simulink model "code_gen_HeadingHold"  (Simulink 7.5)
settings: Solver=FixedStepDiscrete  SolverMode=SingleTasking  StartTime=0.0  StopTime=10.0  FixedStep=0.01  RelTol=1e-3
InitFcn:
  | boat_constants
values from neighbouring files (symbols this model uses):
  figure8_waypoints = int32([ ... (first row only)    [boat_constants.m]
  OC2max = 49999    [boat_constants.m]    (also in simulation_constants.m)
  sampling_waypoints = int32([ ... (first row only)    [boat_constants.m]
  T_step = 0.01    [boat_constants.m]    (also in common.m)
  test_waypoints = int32([ ... (first row only)    [boat_constants.m]
undefined symbols (not defined in the file or in its folder): clearGpsData, clearSensorData, cpInitCommunications, DataEEInitAndClear, DataEEWrite, DiscIntNeverNeededParam, ecan1_buffered_transmit_matlab, ecan1_error_status_matlab, ecan1_init, ecan1_receive_matlab, getGpsData, getSensorData, Init_onlyOnce, Init_Reset, initCalibrationRange, initGps, processNewCommData, processNewGpsData, setHilMode, u1, u2, uart1EnqueueStateData, uart2EnqueueActuatorData, y1
libraries: simulink x85, dsPICdrivers x44, uSimLib x6, simulink_need_slupdate x4, aerolibconvert2 x2
(part 4 of 6)

== system code_gen_HeadingHold/Controller/Radio Control Inputs1/If Action Subsystem5 ==
  input : Inport  OutDataType=fixdt(1, 16)  OutScaling=2^0
  range : Inport  Port=2  OutDataType=fixdt(1, 16)  OutScaling=2^0
  Action Port : ActionPort  ActionType=else
  Add 8% center deadband : Subsystem
  Constant : Constant  Value=0  OutDataType=fixdt(1, 16)  OutScaling=2^0  OutDataTypeStr=Inherit: Inherit via back propagation
  Constant1 : Constant  Value=1000  OutDataType=fixdt(1, 16)  OutScaling=2^0  OutDataTypeStr=Inherit: Inherit via back propagation
  Data Type Conversion : DataTypeConversion  OutDataType=fixdt(1, 16)  OutScaling=2^0
  Data Type Conversion1 : DataTypeConversion  OutDataType=fixdt(1, 16)  OutScaling=2^0
  Demux : Demux  Outputs=2
  Map into range : Stateflow chart  TreatAsAtomicUnit=on
  Saturation : Saturate  UpperLimit=1000  LowerLimit=0  OutDataTypeMode=int16  OutDataType=fixdt(1, 16)  OutScaling=2^0  OutDataTypeStr=int16  RndMeth=Simplest
  Out1 : Outport  OutDataType=fixdt(1, 16)  OutScaling=2^0  InitialOutput=50
  wires:
  Constant1/1 -> Map into range/5(out_max)
  Constant/1 -> Map into range/4(out_min)
  Demux/1 -> Map into range/2(in_min)
  Demux/2 -> Map into range/3(in_max)
  range/1 -> Data Type Conversion1/1
  Map into range/1(mappedValue) -> Saturation/1
  Data Type Conversion/1 -> Map into range/1(val)
  Data Type Conversion1/1 -> Demux/1
  Saturation/1 -> Add 8% center deadband/1(In1)
  input/1 -> Data Type Conversion/1
  Add 8% center deadband/1(Out1) -> Out1/1

== system code_gen_HeadingHold/Controller/Radio Control Inputs1/Reset calibration range ==
  note: Reset the calibration range for each
      | channel before recalibration.
  Trigger : TriggerPort
  Constant1 : Constant  Value=[8000 8000]  OutDataType=fixdt(1, 16)  OutScaling=2^0  OutDataTypeStr=Inherit: Inherit via back propagation  SampleTime=Inf
  Data Store Write : DataStoreWrite  DataStoreName=throttleRange  SampleTime=-1
  Data Store Write1 : DataStoreWrite  DataStoreName=rudderRange  SampleTime=-1
  Data Store Write2 : DataStoreWrite  DataStoreName=trackRange  SampleTime=-1
  wires:
  Constant1/1 -> Data Store Write/1, Data Store Write1/1, Data Store Write2/1

== system code_gen_HeadingHold/Controller/Split trackCommand to singular commands/Countdown timer for trigger ==
  note: calibrationState is a uint8 with 3 states:
      | 0 is off,
      | 1 is timing down waiting to transition,
      | 2 is after a successful transition
  in : Inport
  Constant1 : Constant  OutDataTypeMode=uint8  OutDataType=fixdt(1, 16)  OutScaling=2^0  OutDataTypeStr=uint8  SampleTime=T_step
  Data Store Memory : DataStoreMemory  DataStoreName=timerState  ReadBeforeWriteMsg=warning  WriteAfterWriteMsg=warning  WriteAfterReadMsg=warning  DataType=uint8  OutDataType=fixdt(1, 16)  OutScaling=2^0  OutDataTypeStr=uint8
  Data Store Read : DataStoreRead  DataStoreName=timerState  SampleTime=T_step
  Data Type Conversion1 : DataTypeConversion  OutDataTypeMode=uint8  OutDataType=fixdt(1, 16)  OutScaling=2^0  OutDataTypeStr=uint8
  State transitions : Subsystem
  Timer : DiscreteIntegrator  gainval=100  ExternalReset=level  InitialConditionMode=State only (most efficient)  SampleTime=T_step  OutDataTypeMode=uint8  OutDataType=fixdt(1, 16)  OutScaling=2^0  OutDataTypeStr=uint8  RndMeth=Simplest  LimitOutput=on  UpperSaturationLimit=127  LowerSaturationLimit=0  ICPrevOutput=DiscIntNeverNeededParam  ICPrevScaledInput=DiscIntNeverNeededParam
  Unit Delay2 : UnitDelay  SampleTime=-1
  trigger : Outport  OutDataType=fixdt(1, 16)  OutScaling=2^0
  wires:
  Constant1/1 -> Timer/1
  Timer/1 -> State transitions/1(timer)
  Data Store Read/1 -> State transitions/3(timerState)
  Unit Delay2/1 -> Timer/2
  State transitions/1(startTimer) -> Unit Delay2/1
  in/1 -> Data Type Conversion1/1
  Data Type Conversion1/1 -> State transitions/2(level)
  State transitions/2(trigger) -> trigger/1

== system code_gen_HeadingHold/Controller/Split trackCommand to singular commands/Countdown timer for trigger1 ==
  note: calibrationState is a uint8 with 3 states:
      | 0 is off,
      | 1 is timing down waiting to transition,
      | 2 is after a successful transition
  in : Inport
  Constant1 : Constant  OutDataTypeMode=uint8  OutDataType=fixdt(1, 16)  OutScaling=2^0  OutDataTypeStr=uint8  SampleTime=T_step
  Data Store Memory : DataStoreMemory  DataStoreName=timerState2  ReadBeforeWriteMsg=warning  WriteAfterWriteMsg=warning  WriteAfterReadMsg=warning  DataType=uint8  OutDataType=fixdt(1, 16)  OutScaling=2^0  OutDataTypeStr=uint8
  Data Store Read : DataStoreRead  DataStoreName=timerState2  SampleTime=T_step
  Data Type Conversion1 : DataTypeConversion  OutDataTypeMode=uint8  OutDataType=fixdt(1, 16)  OutScaling=2^0  OutDataTypeStr=uint8
  State transitions : Subsystem
  Timer : DiscreteIntegrator  gainval=100  ExternalReset=level  InitialConditionMode=State only (most efficient)  SampleTime=T_step  OutDataTypeMode=uint8  OutDataType=fixdt(1, 16)  OutScaling=2^0  OutDataTypeStr=uint8  RndMeth=Simplest  LimitOutput=on  UpperSaturationLimit=127  LowerSaturationLimit=0  ICPrevOutput=DiscIntNeverNeededParam  ICPrevScaledInput=DiscIntNeverNeededParam
  Unit Delay2 : UnitDelay  SampleTime=-1
  trigger : Outport  OutDataType=fixdt(1, 16)  OutScaling=2^0
  wires:
  State transitions/2(trigger) -> trigger/1
  Data Type Conversion1/1 -> State transitions/2(level)
  in/1 -> Data Type Conversion1/1
  State transitions/1(startTimer) -> Unit Delay2/1
  Unit Delay2/1 -> Timer/2
  Data Store Read/1 -> State transitions/3(timerState)
  Timer/1 -> State transitions/1(timer)
  Constant1/1 -> Timer/1

== system code_gen_HeadingHold/Sensor Inputs/Estop detection/If Action Subsystem ==
  data : Inport  OutDataType=fixdt(1, 16)  OutScaling=2^0
  Action Port : ActionPort  ActionType=then
  Bitwise Operator : simulink/Logic and Bit Operations/Bitwise Operator  logicop=OR  UseBitMask=off  NumInputPorts=2  BitMask=bin2dec('11011001')  BitMaskRealWorld=Stored Integer
  Data Store Write : DataStoreWrite  DataStoreName=v_rpm  SampleTime=-1
  Data Type Conversion2 : DataTypeConversion  OutDataTypeMode=int16  OutDataType=fixdt(1, 16)  OutScaling=2^0  OutDataTypeStr=int16
  Data Type Conversion3 : DataTypeConversion  OutDataTypeMode=uint16  OutDataType=fixdt(1, 16)  OutScaling=2^0  OutDataTypeStr=uint16
  Demux : Demux  Outputs=2
  Selector : Selector  InputPortWidth=8  IndexOptions=Index vector (dialog)  Indices=[1 2]  OutputSizes=1
  Shift Arithmetic : simulink/Logic and Bit Operations/Shift Arithmetic  SystemSampleTime=-1  nBitShiftRight=-8  nBinPtShiftRight=0
  wires:
  Demux/1 -> Shift Arithmetic/1
  Shift Arithmetic/1 -> Bitwise Operator/1
  Demux/2 -> Bitwise Operator/2
  Selector/1 -> Data Type Conversion3/1
  Bitwise Operator/1 -> Data Type Conversion2/1
  data/1 -> Selector/1
  Data Type Conversion2/1 -> Data Store Write/1
  Data Type Conversion3/1 -> Demux/1

== system code_gen_HeadingHold/Sensor Inputs/Estop detection/Receive ECAN1 Message ==
  C Function Call [ecanFunctions.c] : dsPICdrivers/OTHERS/C Function Call  Tag=dsPIC_dsPIC_CFunctionCall  FctUpdate=Output Function  fctName='ecan1_receive_matlab'  INPUT_SIZE=1  INPUT1=--  INPUT2=--  INPUT3=--  OUTPUT_SIZE=4  OUTPUT1=uint32  SampleTime=ecan1_receive_sample_time  InputType=[ ]  OutputType=[ 6 ]  FctDeclaration=extern void ecan1_receive_matlab(uint32_T* y1);  FctCall=ecan1_receive_matlab(*%y1);  OrderingInOutPopup=None  FctStart=None  FctStart_Name=Init_onlyOnce  FctStart_Declaration=inline extern void Init_onlyOnce();  FctStart_Call=Init_onlyOnce();  FctInit=None  FctInit_Name=Init_Reset  FctInit_Declaration=inline extern void Init_Reset();  FctInit_Call=Init_Reset();  PinDigitalInput=[]  PinDigitalOutput=[]  AnalogueInput=[]
  Compare To Zero : simulink/Logic and Bit Operations/Compare To Zero  SystemSampleTime=-1  relop=~=  LogicOutDataTypeMode=uint8  ZeroCross=off
  Data Type Conversion : DataTypeConversion  OutDataTypeMode=boolean  OutDataType=sfix(16)  OutScaling=2^0  OutDataTypeStr=boolean
  Data Type Conversion1 : DataTypeConversion  OutDataTypeMode=uint32  OutDataType=fixdt(1, 16)  OutScaling=2^0  OutDataTypeStr=uint32
  Decompose uint64 : Subsystem
  Demux : Demux
  Extract Bits : simulink/Logic and Bit Operations/Extract Bits  SystemSampleTime=-1  bitsToExtract=Lower half  numBits=8  bitIdxRange=[0 7]  outScalingMode=Treat bit field as an integer
  Extract Bits1 : simulink/Logic and Bit Operations/Extract Bits  SystemSampleTime=-1  bitsToExtract=Range of bits  numBits=8  bitIdxRange=[16 23]  outScalingMode=Treat bit field as an integer
  Extract Bits2 : simulink/Logic and Bit Operations/Extract Bits  SystemSampleTime=-1  bitsToExtract=Range ending with least significant bit  numBits=29  bitIdxRange=[0 7]  outScalingMode=Treat bit field as an integer
  identifier : Outport  OutDataType=sfix(16)  OutScaling=2^0
  data : Outport  Port=2  OutDataType=sfix(16)  OutScaling=2^0
  remote : Outport  Port=3  OutDataType=sfix(16)  OutScaling=2^0
  new : Outport  Port=4  OutDataType=sfix(16)  OutScaling=2^0
  size : Outport  Port=5  OutDataType=sfix(16)  OutScaling=2^0
  wires:
  C Function Call [ecanFunctions.c]/1 -> Demux/1
  Demux/1 -> Extract Bits2/1, Compare To Zero/1
  Demux/3 -> Decompose uint64/2(high-order uint1)
  Demux/4 -> Extract Bits/1, Extract Bits1/1
  Data Type Conversion/1 -> remote/1
  Demux/2 -> Decompose uint64/1(low-order uint32)
  Extract Bits/1 -> Data Type Conversion/1
  Decompose uint64/1(uint8 array) -> data/1
  Extract Bits2/1 -> Data Type Conversion1/1
  Compare To Zero/1 -> new/1
  Extract Bits1/1 -> size/1
  Data Type Conversion1/1 -> identifier/1

== system code_gen_HeadingHold/Transmit actuator data/Package and Transmit Sensor Struct/Build HIL sentence ==
  data : Inport
  Bitwise Operator : simulink/Logic and Bit Operations/Bitwise Operator  logicop=XOR  UseBitMask=off  BitMask=bin2dec('11011001')  BitMaskRealWorld=Stored Integer
  Constant : Constant  Value=37  OutDataTypeMode=uint8  OutDataType=fixdt(1, 16)  OutScaling=2^0  OutDataTypeStr=uint8
  Constant1 : Constant  Value=38  OutDataTypeMode=uint8  OutDataType=fixdt(1, 16)  OutScaling=2^0  OutDataTypeStr=uint8
  Constant2 : Constant  Value=94  OutDataTypeMode=uint8  OutDataType=fixdt(1, 16)  OutScaling=2^0  OutDataTypeStr=uint8
  Constant3 : Constant  Value=38  OutDataTypeMode=uint8  OutDataType=fixdt(1, 16)  OutScaling=2^0  OutDataTypeStr=uint8
  Constant4 : Constant  Value=2  OutDataTypeMode=uint8  OutDataType=fixdt(1, 16)  OutScaling=2^0  OutDataTypeStr=uint8
  Mux2 : Mux  Inputs=3
  Pack : Stateflow chart  TreatAsAtomicUnit=on
  Probe : Probe  ProbeSampleTime=off  ProbeComplexSignal=off  ProbeWidthDataType=uint8
  sent : Outport
  wires:
  data/1 -> Probe/1, Mux2/3
  Constant/1 -> Pack/1(a)
  Constant1/1 -> Pack/2(b)
  Pack/1(y) -> sent/1
  Mux2/1 -> Bitwise Operator/1, Pack/3(c)
  Probe/1 -> Mux2/2
  Constant2/1 -> Pack/4(d)
  Constant3/1 -> Pack/5(e)
  Bitwise Operator/1 -> Pack/6(f)
  Constant4/1 -> Mux2/1

== system code_gen_HeadingHold/Controller/Auto/Manual Switch/Rudder calibration controller/Rudder Command ==
  note: Up and period are both defined to generate a 50% duty cycle PWM with
      | a period of 3ms.
  step : Inport
  dir : Inport  Port=2
  Bus Creator : BusCreator
  Constant1 : Constant  Value=.003*OC2max/.01  OutDataTypeMode=uint16  OutDataType=sfix(16)  OutScaling=2^0  OutDataTypeStr=uint16
  Constant3 : Constant  Value=0  OutDataTypeMode=boolean  OutDataType=sfix(16)  OutScaling=2^0  OutDataTypeStr=boolean
  Constant4 : Constant  Value=0  OutDataTypeMode=uint16  OutDataType=sfix(16)  OutScaling=2^0  OutDataTypeStr=uint16
  Shift Arithmetic : simulink/Logic and Bit Operations/Shift Arithmetic  SystemSampleTime=-1  nBitShiftRight=1  nBinPtShiftRight=0
  Switch : Switch  Criteria=u2 ~= 0  OutDataType=fixdt(1, 16)  OutScaling=2^0
  Switch1 : Switch  Criteria=u2 ~= 0  OutDataType=fixdt(1, 16)  OutScaling=2^0
  Command : Outport
  wires:
  step/1 -> Switch1/2, Switch/2
  Constant4/1 -> Switch1/3, Switch/3
  Switch1/1 -> Bus Creator/3  "up"
  Switch/1 -> Bus Creator/4  "period"
  Shift Arithmetic/1 -> Switch1/1
  Constant1/1 -> Switch/1, Shift Arithmetic/1
  Constant3/1 -> Bus Creator/1  "enable"
  Bus Creator/1 -> Command/1
  dir/1 -> Bus Creator/2  "direction"

== system code_gen_HeadingHold/Controller/Auto/Manual Switch/Rudder calibration controller/Throttle Command ==
  en : Inport
  Bus Creator : BusCreator
  Logical Operator : Logic  Operator=NOT  AllPortsSameDT=off  OutDataTypeMode=boolean  LogicDataType=fixdt(0, 8)  OutDataTypeStr=boolean
  Mux Everything : Subsystem
  command : Outport  OutDataType=sfix(16)  OutScaling=2^0
  wires:
  Mux Everything/3(size) -> Bus Creator/3  "size"
  Mux Everything/2(data) -> Bus Creator/2  "data"
  Mux Everything/1(iden) -> Bus Creator/1  "identifier"
  en/1 -> Logical Operator/1
  Bus Creator/1 -> command/1
  Logical Operator/1 -> Mux Everything/1(reset)
  Mux Everything/4(trig) -> Bus Creator/4  "trigger"

== system code_gen_HeadingHold/Controller/Autonomous Controller/Rudder Command/Heading Control ==
  note: Heading Error
  V_boat [m/s] : Inport  OutDataType=sfix(16)  OutScaling=2^0
  Psi desired [deg] : Inport  Port=2  OutDataType=sfix(16)  OutScaling=2^0
  Heading [deg] : Inport  Port=3  OutDataType=sfix(16)  OutScaling=2^0
  CrossTrack Error [m] : Inport  Port=4  OutDataType=sfix(16)  OutScaling=2^0
  Abs : Abs
  Angle Conversion : aerolibconvert2/Angle Conversion  SystemSampleTime=-1  IU=deg  OU=rad
  Angle Conversion1 : aerolibconvert2/Angle Conversion  SystemSampleTime=-1  IU=rad  OU=deg
  Constant : Constant  OutDataType=sfix(16)  OutScaling=2^0
  Divide : Product  Inputs=*/  OutDataType=sfix(16)  OutScaling=2^-10
  Fcn2 : Fcn  Expr=(u<-180)*360 + u + (u>180)*(-360)
  Kpsi : Gain  ParameterDataType=sfix(16)  ParameterScaling=2^0  OutDataType=sfix(16)  OutScaling=2^0
  MinMax : MinMax  Function=max  Inputs=2  OutDataType=sfix(16)  OutScaling=2^0
  Product : Product  OutDataType=sfix(16)  OutScaling=2^0  RndMeth=Zero
  Saturation : Saturate  UpperLimit=45  LowerLimit=-45
  Scope : Scope
      settings: SaveName=ScopeData4
  Sign : Signum
  Sum : Sum  Inputs=-+|  OutDataType=sfix(16)  OutScaling=2^0
  Terminator : Terminator
  delta_R [deg] : Outport  OutDataType=sfix(16)  OutScaling=2^0
  wires:
  Fcn2/1 -> Angle Conversion/1, Scope/1
  Angle Conversion/1 -> Kpsi/1
  V_boat [m/s]/1 -> Abs/1, Sign/1
  Product/1 -> Angle Conversion1/1
  Kpsi/1 -> Product/2
  Sign/1 -> Product/1
  Angle Conversion1/1 -> Divide/1
  Divide/1 -> Saturation/1
  Abs/1 -> MinMax/1
  Constant/1 -> MinMax/2
  Saturation/1 -> delta_R [deg]/1
  MinMax/1 -> Divide/2
  CrossTrack Error [m]/1 -> Terminator/1
  Psi desired [deg]/1 -> Sum/1
  Heading [deg]/1 -> Sum/2
  Sum/1 -> Fcn2/1

== system code_gen_HeadingHold/Controller/Autonomous Controller/State Keeper & Estimator/Ballast Estimator ==
  b : Inport
  Bus Selector1 : BusSelector  OutputSignals=position
  sensors_b : Outport
  wires:
  Bus Selector1/1 -> sensors_b/1  "<position>"
  b/1 -> Bus Selector1/1

== system code_gen_HeadingHold/Controller/Autonomous Controller/State Keeper & Estimator/GPS Estimator ==
  gps : Inport
  reset : Inport  Port=2  OutDataType=fixdt(1, 16)  OutScaling=2^0
  Add : Sum  OutDataType=fixdt(1, 16)  OutScaling=2^-10
  Bus Selector1 : BusSelector  OutputSignals=latitude,longitude,altitude,newData
  Calculate local position via velocity integral between true GPS updates : Stateflow chart  TreatAsAtomicUnit=on
  Discrete-Time Integrator4 : DiscreteIntegrator  ExternalReset=level  SampleTime=-1  OutDataType=fixdt(1, 16)  OutScaling=2^0  ICPrevOutput=DiscIntNeverNeededParam  ICPrevScaledInput=DiscIntNeverNeededParam
  Mux1 : Mux  Inputs=3
  Subsystem : Subsystem
  velocity : Outport
  pos : Outport  Port=2
  heading : Outport  Port=3
  lla : Outport  Port=4
  datetime : Outport  Port=5
  wires:
  Subsystem/1(velocity) -> velocity/1, Discrete-Time Integrator4/1
  Calculate local position via velocity integral between true GPS updates/1(localPosition) -> Add/1
  Calculate local position via velocity integral between true GPS updates/2(resetIntegrator) -> Discrete-Time Integrator4/2
  Mux1/1 -> Calculate local position via velocity integral between true GPS updates/1(latLonAlt)
  Bus Selector1/4 -> Calculate local position via velocity integral between true GPS updates/2(newData)  "<newData>"
  Bus Selector1/3 -> Mux1/3  "<altitude>"
  Bus Selector1/2 -> Mux1/2  "<longitude>"
  Bus Selector1/1 -> Mux1/1  "<latitude>"
  Add/1 -> pos/1
  Discrete-Time Integrator4/1 -> Add/2
  reset/1 -> Calculate local position via velocity integral between true GPS updates/3(reset)
  Subsystem/4(time) -> datetime/1
  Subsystem/3(pos) -> lla/1
  gps/1 -> Bus Selector1/1, Subsystem/1(gps)
  Subsystem/2(heading) -> heading/1

== system code_gen_HeadingHold/Controller/Autonomous Controller/State Keeper & Estimator/Rudder Estimator ==
  r : Inport
  sensors_r : Outport
  wires:
  r/1 -> sensors_r/1

== system code_gen_HeadingHold/Controller/Autonomous Controller/State Keeper & Estimator/Throttle Estimator ==
  t : Inport
  sensors_t : Outport
  wires:
  t/1 -> sensors_t/1

== system code_gen_HeadingHold/Controller/Autonomous Controller/Throttle Command/Mux Everything ==
  speed : Inport  OutDataType=sfix(16)  OutScaling=2^0
  disable : Inport  Port=2  OutDataType=sfix(16)  OutScaling=2^0
  enable : Inport  Port=3  OutDataType=sfix(16)  OutScaling=2^0
  Throttle : Inport  Port=4  OutDataType=sfix(16)  OutScaling=2^0
  0x300 : Constant  Value=768  OutDataTypeMode=uint32  OutDataType=sfix(16)  OutScaling=2^0  OutDataTypeStr=uint32
  0x301 : Constant  Value=769  OutDataTypeMode=uint32  OutDataType=sfix(16)  OutScaling=2^0  OutDataTypeStr=uint32
  Build speed command : Subsystem
  Disable motor : Constant  Value=[0 0 0 0 64 0]  OutDataTypeMode=uint8  OutDataType=sfix(16)  OutScaling=2^0  OutDataTypeStr=uint8
  Enable motor : Constant  Value=[0 0 0 0 32 0]  OutDataTypeMode=uint8  OutDataType=sfix(16)  OutScaling=2^0  OutDataTypeStr=uint8
  Logical Operator1 : Logic  Operator=OR  AllPortsSameDT=off  OutDataTypeMode=boolean  OutDataTypeStr=boolean
  Message Length1 : Probe  ProbeSampleTime=off  ProbeComplexSignal=off  ProbeWidthDataType=uint8
  Multiport Switch : MultiPortSwitch  zeroidx=off
  Multiport Switch1 : MultiPortSwitch  zeroidx=off
  Select data packet : Stateflow chart  TreatAsAtomicUnit=on
  Switch : Switch  Criteria=u2 ~= 0
  iden : Outport  OutDataType=sfix(16)  OutScaling=2^0
  data : Outport  Port=2  OutDataType=sfix(16)  OutScaling=2^0
  size : Outport  Port=3  OutDataType=sfix(16)  OutScaling=2^0
  trig : Outport  Port=4  OutDataType=sfix(16)  OutScaling=2^0
  wires:
  Build speed command/1(msg) -> Multiport Switch/4
  speed/1 -> Multiport Switch1/4
  Multiport Switch1/1 -> trig/1
  Select data packet/1(y) -> Multiport Switch1/1, Multiport Switch/1
  Logical Operator1/1 -> Switch/2
  enable/1 -> Multiport Switch1/3, Select data packet/2(en), Logical Operator1/2
  disable/1 -> Multiport Switch1/2, Select data packet/1(dis), Logical Operator1/1
  Switch/1 -> iden/1
  0x301/1 -> Switch/3
  0x300/1 -> Switch/1
  Message Length1/1 -> size/1
  Multiport Switch/1 -> data/1, Message Length1/1
  Throttle/1 -> Build speed command/1(CC)
  Disable motor/1 -> Multiport Switch/2
  Enable motor/1 -> Multiport Switch/3

== system code_gen_HeadingHold/Controller/Autonomous Controller/Throttle Command/Trigger Events ==
  RC Throttle : Inport  OutDataType=sfix(16)  OutScaling=2^0
  Reset : Inport  Port=2  OutDataType=sfix(16)  OutScaling=2^0
  Data Type Conversion1 : DataTypeConversion  OutDataTypeMode=boolean  OutDataType=sfix(16)  OutScaling=2^0  OutDataTypeStr=boolean
  Data Type Conversion2 : DataTypeConversion  OutDataTypeMode=boolean  OutDataType=sfix(16)  OutScaling=2^0  OutDataTypeStr=boolean
  Data Type Conversion3 : DataTypeConversion  OutDataTypeMode=boolean  OutDataType=sfix(16)  OutScaling=2^0  OutDataTypeStr=boolean
  Detect Change : simulink/Logic and Bit Operations/Detect Change  SystemSampleTime=-1  vinit=0
  Detect Fall Nonpositive : simulink/Logic and Bit Operations/Detect Fall Nonpositive  SystemSampleTime=-1  vinit=0
  Detect Rise Positive : simulink/Logic and Bit Operations/Detect Rise Positive  SystemSampleTime=-1  vinit=0
  Shift Arithmetic : simulink/Logic and Bit Operations/Shift Arithmetic  SystemSampleTime=-1  nBitShiftRight=2  nBinPtShiftRight=0
  Weighted Moving Average : simulink_need_slupdate/Weighted Moving Average  mgainval=[.5 .5]  vinit=0.0  samptime=-1  OutDataTypeStr=Inherit: Inherit via back propagation  OutDataType=sfix(16)  OutScaling=2^-10  DoSatur=off  GainDataType=uint(16)  MatRadixGroup=Best Precision: Matrix-wise  GainScaling=2^-10
  Change Speed : Outport  OutDataType=sfix(16)  OutScaling=2^0
  Disable : Outport  Port=2  OutDataType=sfix(16)  OutScaling=2^0
  Enable : Outport  Port=3  OutDataType=sfix(16)  OutScaling=2^0
  wires:
  Data Type Conversion1/1 -> Disable/1
  Data Type Conversion2/1 -> Enable/1
  Data Type Conversion3/1 -> Change Speed/1
  Detect Rise Positive/1 -> Data Type Conversion1/1
  Detect Fall Nonpositive/1 -> Data Type Conversion2/1
  Reset/1 -> Detect Rise Positive/1, Detect Fall Nonpositive/1
  Shift Arithmetic/1 -> Weighted Moving Average/1
  Weighted Moving Average/1 -> Detect Change/1
  Detect Change/1 -> Data Type Conversion3/1
  RC Throttle/1 -> Shift Arithmetic/1

== system code_gen_HeadingHold/Controller/RC Inputs/Map PWM values to Actuator Signals/Manual Rudder Command ==
  note: This subsystem wraps the RC rudder command inside a proportional controller. It follows the same
      | logic used within the Autonomous Controller.
  note: Enable is an active-low signal for the 2035
      | driver board currently being used.
  RC Rudder : Inport  OutDataType=sfix(16)  OutScaling=2^0
  rudderAngle : Inport  Port=2  OutDataType=sfix(16)  OutScaling=2^0
  Abs : Abs  OutDataType=fixdt(1, 16)  OutScaling=2^0
  Add : Sum  Inputs=-+  OutDataType=fixdt(1, 16)  OutScaling=2^-10
  Bus Creator1 : BusCreator
  Compare To Constant : simulink/Logic and Bit Operations/Compare To Constant  SystemSampleTime=-1  relop=>  const=.03  LogicOutDataTypeMode=boolean
  Constant3 : Constant  Value=.003*OC2max/.01  OutDataTypeMode=uint16  OutDataType=sfix(16)  OutScaling=2^0  OutDataTypeStr=uint16
  Constant5 : Constant  Value=0  OutDataTypeMode=boolean  OutDataType=sfix(16)  OutScaling=2^0  OutDataTypeStr=boolean
  Constant6 : Constant  Value=0  OutDataTypeMode=uint16  OutDataType=sfix(16)  OutScaling=2^0  OutDataTypeStr=uint16
  Data Type Conversion : DataTypeConversion  OutDataTypeMode=boolean  OutDataType=fixdt(1, 16)  OutScaling=2^0  OutDataTypeStr=boolean  RndMeth=Simplest
  Saturation1 : Saturate  UpperLimit=1  LowerLimit=0  OutDataTypeStr=Inherit: Inherit via back propagation
  Shift Arithmetic1 : simulink/Logic and Bit Operations/Shift Arithmetic  SystemSampleTime=-1  nBitShiftRight=1  nBinPtShiftRight=0
  Sign : Signum
  Switch2 : Switch  Criteria=u2 ~= 0  OutDataType=fixdt(1, 16)  OutScaling=2^0
  Switch3 : Switch  Criteria=u2 ~= 0  OutDataType=fixdt(1, 16)  OutScaling=2^0
  Rudder Command : Outport
  wires:
  RC Rudder/1 -> Add/2
  Bus Creator1/1 -> Rudder Command/1
  Add/1 -> Abs/1, Sign/1
  Compare To Constant/1 -> Switch3/2, Switch2/2
  Constant6/1 -> Switch3/3, Switch2/3
  Switch3/1 -> Bus Creator1/3  "up"
  Switch2/1 -> Bus Creator1/4  "period"
  Shift Arithmetic1/1 -> Switch3/1
  Abs/1 -> Compare To Constant/1
  Constant3/1 -> Switch2/1, Shift Arithmetic1/1
  Constant5/1 -> Bus Creator1/1  "enable"
  Sign/1 -> Saturation1/1
  Saturation1/1 -> Data Type Conversion/1
  Data Type Conversion/1 -> Bus Creator1/2  "direction"
  rudderAngle/1 -> Add/1

== system code_gen_HeadingHold/Controller/RC Inputs/Map PWM values to Actuator Signals/Throttle Command ==
  speed : Inport
  Bus Creator : BusCreator
  Detect Rise Positive : simulink/Logic and Bit Operations/Detect Rise Positive  SystemSampleTime=-1  vinit=0
  Mux Everything : Subsystem
  Trigger Events : Subsystem
  command : Outport  OutDataType=sfix(16)  OutScaling=2^0
  wires:
  Bus Creator/1 -> command/1
  speed/1 -> Trigger Events/1(Throttle), Detect Rise Positive/1, Mux Everything/3(Throttle)
  Mux Everything/1(iden) -> Bus Creator/1  "identifier"
  Mux Everything/3(size) -> Bus Creator/3  "size"
  Mux Everything/4(trig) -> Bus Creator/4  "trigger"
  Mux Everything/2(data) -> Bus Creator/2  "data"
  Trigger Events/1(Change Speed) -> Mux Everything/1(speed)
  Detect Rise Positive/1 -> Mux Everything/2(enable)

== system code_gen_HeadingHold/Controller/Radio Control Inputs1/Calibration/Store rudder range to memory ==
  rudderRange : Inport
  Constant : Constant  Value=11  OutDataType=fixdt(1, 16)  OutScaling=2^0  OutDataTypeStr=Inherit: Inherit via back propagation
  Constant1 : Constant  Value=10  OutDataType=fixdt(1, 16)  OutScaling=2^0  OutDataTypeStr=Inherit: Inherit via back propagation
  Demux : Demux  Outputs=2
  Store rudder range  maximum to memory [DEE.c] : dsPICdrivers/OTHERS/C Function Call  Tag=dsPIC_dsPIC_CFunctionCall  FctUpdate=Output Function  fctName='DataEEWrite'  INPUT_SIZE=1  INPUT1=uint16  INPUT2=uint8  INPUT3=--  OUTPUT_SIZE=1  OUTPUT1=--  SampleTime=T_step  InputType=[ 4 2 ]  OutputType=[ ]  FctDeclaration=extern void DataEEWrite(uint16_T u1, uint8_T u2);  FctCall=DataEEWrite(%u1, %u2);  OrderingInOutPopup=None  FctStart=None  FctStart_Name=Init_onlyOnce  FctStart_Declaration=inline extern void Init_onlyOnce();  FctStart_Call=Init_onlyOnce();  FctInit=None  FctInit_Name=Init_Reset  FctInit_Declaration=inline extern void Init_Reset();  FctInit_Call=Init_Reset();  PinDigitalInput=[]  PinDigitalOutput=[]  AnalogueInput=[]
  Store rudder range  minimum to memory [DEE.c] : dsPICdrivers/OTHERS/C Function Call  Tag=dsPIC_dsPIC_CFunctionCall  FctUpdate=Output Function  fctName='DataEEWrite'  INPUT_SIZE=1  INPUT1=uint16  INPUT2=uint8  INPUT3=--  OUTPUT_SIZE=1  OUTPUT1=--  SampleTime=T_step  InputType=[ 4 2 ]  OutputType=[ ]  FctDeclaration=extern void DataEEWrite(uint16_T u1, uint8_T u2);  FctCall=DataEEWrite(%u1, %u2);  OrderingInOutPopup=None  FctStart=None  FctStart_Name=Init_onlyOnce  FctStart_Declaration=inline extern void Init_onlyOnce();  FctStart_Call=Init_onlyOnce();  FctInit=None  FctInit_Name=Init_Reset  FctInit_Declaration=inline extern void Init_Reset();  FctInit_Call=Init_Reset();  PinDigitalInput=[]  PinDigitalOutput=[]  AnalogueInput=[]
  wires:
  Demux/2 -> Store rudder range  maximum to memory [DEE.c]/1
  Demux/1 -> Store rudder range  minimum to memory [DEE.c]/1
  Constant/1 -> Store rudder range  maximum to memory [DEE.c]/2
  Constant1/1 -> Store rudder range  minimum to memory [DEE.c]/2
  rudderRange/1 -> Demux/1

== system code_gen_HeadingHold/Controller/Radio Control Inputs1/Calibration/Store throttle range to memory ==
  throttleRange : Inport
  Constant : Constant  Value=13  OutDataType=fixdt(1, 16)  OutScaling=2^0  OutDataTypeStr=Inherit: Inherit via back propagation
  Constant1 : Constant  Value=12  OutDataType=fixdt(1, 16)  OutScaling=2^0  OutDataTypeStr=Inherit: Inherit via back propagation
  Demux : Demux  Outputs=2
  Store throttle range  maximum to memory [DEE.c] : dsPICdrivers/OTHERS/C Function Call  Tag=dsPIC_dsPIC_CFunctionCall  FctUpdate=Output Function  fctName='DataEEWrite'  INPUT_SIZE=1  INPUT1=uint16  INPUT2=uint8  INPUT3=--  OUTPUT_SIZE=1  OUTPUT1=--  SampleTime=T_step  InputType=[ 4 2 ]  OutputType=[ ]  FctDeclaration=extern void DataEEWrite(uint16_T u1, uint8_T u2);  FctCall=DataEEWrite(%u1, %u2);  OrderingInOutPopup=None  FctStart=None  FctStart_Name=Init_onlyOnce  FctStart_Declaration=inline extern void Init_onlyOnce();  FctStart_Call=Init_onlyOnce();  FctInit=None  FctInit_Name=Init_Reset  FctInit_Declaration=inline extern void Init_Reset();  FctInit_Call=Init_Reset();  PinDigitalInput=[]  PinDigitalOutput=[]  AnalogueInput=[]
  Store throttle range  minimum to memory [DEE.c] : dsPICdrivers/OTHERS/C Function Call  Tag=dsPIC_dsPIC_CFunctionCall  FctUpdate=Output Function  fctName='DataEEWrite'  INPUT_SIZE=1  INPUT1=uint16  INPUT2=uint8  INPUT3=--  OUTPUT_SIZE=1  OUTPUT1=--  SampleTime=T_step  InputType=[ 4 2 ]  OutputType=[ ]  FctDeclaration=extern void DataEEWrite(uint16_T u1, uint8_T u2);  FctCall=DataEEWrite(%u1, %u2);  OrderingInOutPopup=None  FctStart=None  FctStart_Name=Init_onlyOnce  FctStart_Declaration=inline extern void Init_onlyOnce();  FctStart_Call=Init_onlyOnce();  FctInit=None  FctInit_Name=Init_Reset  FctInit_Declaration=inline extern void Init_Reset();  FctInit_Call=Init_Reset();  PinDigitalInput=[]  PinDigitalOutput=[]  AnalogueInput=[]
  wires:
  Demux/2 -> Store throttle range  maximum to memory [DEE.c]/1
  Demux/1 -> Store throttle range  minimum to memory [DEE.c]/1
  Constant/1 -> Store throttle range  maximum to memory [DEE.c]/2
  Constant1/1 -> Store throttle range  minimum to memory [DEE.c]/2
  throttleRange/1 -> Demux/1

== system code_gen_HeadingHold/Controller/Radio Control Inputs1/Calibration/Store track range to memory ==
  trackRange : Inport
  Constant : Constant  Value=15  OutDataType=fixdt(1, 16)  OutScaling=2^0  OutDataTypeStr=Inherit: Inherit via back propagation
  Constant1 : Constant  Value=14  OutDataType=fixdt(1, 16)  OutScaling=2^0  OutDataTypeStr=Inherit: Inherit via back propagation
  Demux : Demux  Outputs=2
  Store track range  maximum to memory [DEE.c] : dsPICdrivers/OTHERS/C Function Call  Tag=dsPIC_dsPIC_CFunctionCall  FctUpdate=Output Function  fctName='DataEEWrite'  INPUT_SIZE=1  INPUT1=uint16  INPUT2=uint8  INPUT3=--  OUTPUT_SIZE=1  OUTPUT1=--  SampleTime=T_step  InputType=[ 4 2 ]  OutputType=[ ]  FctDeclaration=extern void DataEEWrite(uint16_T u1, uint8_T u2);  FctCall=DataEEWrite(%u1, %u2);  OrderingInOutPopup=None  FctStart=None  FctStart_Name=Init_onlyOnce  FctStart_Declaration=inline extern void Init_onlyOnce();  FctStart_Call=Init_onlyOnce();  FctInit=None  FctInit_Name=Init_Reset  FctInit_Declaration=inline extern void Init_Reset();  FctInit_Call=Init_Reset();  PinDigitalInput=[]  PinDigitalOutput=[]  AnalogueInput=[]
  Store track range  minimum to memory [DEE.c] : dsPICdrivers/OTHERS/C Function Call  Tag=dsPIC_dsPIC_CFunctionCall  FctUpdate=Output Function  fctName='DataEEWrite'  INPUT_SIZE=1  INPUT1=uint16  INPUT2=uint8  INPUT3=--  OUTPUT_SIZE=1  OUTPUT1=--  SampleTime=T_step  InputType=[ 4 2 ]  OutputType=[ ]  FctDeclaration=extern void DataEEWrite(uint16_T u1, uint8_T u2);  FctCall=DataEEWrite(%u1, %u2);  OrderingInOutPopup=None  FctStart=None  FctStart_Name=Init_onlyOnce  FctStart_Declaration=inline extern void Init_onlyOnce();  FctStart_Call=Init_onlyOnce();  FctInit=None  FctInit_Name=Init_Reset  FctInit_Declaration=inline extern void Init_Reset();  FctInit_Call=Init_Reset();  PinDigitalInput=[]  PinDigitalOutput=[]  AnalogueInput=[]
  wires:
  Demux/2 -> Store track range  maximum to memory [DEE.c]/1
  Demux/1 -> Store track range  minimum to memory [DEE.c]/1
  Constant/1 -> Store track range  maximum to memory [DEE.c]/2
  Constant1/1 -> Store track range  minimum to memory [DEE.c]/2
  trackRange/1 -> Demux/1

== system code_gen_HeadingHold/Controller/Radio Control Inputs1/Calibration/Update range from input ==
  note: Update lower range limit.
      | The new value is checked against a sane range of 5000-11000
      | to keep values realistic.
  note: Update upper range limit
  limitRange : Inport
  newValue : Inport  Port=2
  If : If  NumInputs=2  IfExpression=u1 < u2 & u1 > 5000 & u1 >= 0
  If Action Subsystem : Subsystem  TreatAsAtomicUnit=on
  If Action Subsystem1 : Subsystem  TreatAsAtomicUnit=on
  If Action Subsystem2 : Subsystem  TreatAsAtomicUnit=on
  If Action Subsystem3 : Subsystem  TreatAsAtomicUnit=on
  If1 : If  NumInputs=2  IfExpression=u1 > u2 & u1 < 11000 & u1 >= 0
  Merge : Merge
  Merge1 : Merge
  Mux : Mux  Inputs=2
  Selector : Selector  InputPortWidth=2  IndexOptions=Index vector (dialog)  Indices=[1]  OutputSizes=1
  Selector1 : Selector  InputPortWidth=2  IndexOptions=Index vector (dialog)  Indices=[2]  OutputSizes=1
  newRange : Outport
  wires:
  Selector/1 -> If/2, If Action Subsystem1/1(In1)
  Selector1/1 -> If Action Subsystem3/1(In1), If1/2
  Mux/1 -> newRange/1
  Merge1/1 -> Mux/2
  Merge/1 -> Mux/1
  If Action Subsystem3/1(Out1) -> Merge1/2
  If Action Subsystem2/1(Out1) -> Merge1/1
  If1/2 -> If Action Subsystem3/Action
  If1/1 -> If Action Subsystem2/Action
  If Action Subsystem1/1(Out1) -> Merge/2
  If Action Subsystem/1(Out1) -> Merge/1
  If/2 -> If Action Subsystem1/Action
  If/1 -> If Action Subsystem/Action
  newValue/1 -> If Action Subsystem/1(In1), If/1, If Action Subsystem2/1(In1), If1/1
  limitRange/1 -> Selector/1, Selector1/1

== system code_gen_HeadingHold/Controller/Radio Control Inputs1/Calibration/Update range from input1 ==
  note: Update lower range limit.
      | The new value is checked against a sane range of 5000-11000
      | to keep values realistic.
  note: Update upper range limit
  limitRange : Inport
  newValue : Inport  Port=2
  If : If  NumInputs=2  IfExpression=u1 < u2 & u1 > 5000 & u1 >= 0
  If Action Subsystem : Subsystem  TreatAsAtomicUnit=on
  If Action Subsystem1 : Subsystem  TreatAsAtomicUnit=on
  If Action Subsystem2 : Subsystem  TreatAsAtomicUnit=on
  If Action Subsystem3 : Subsystem  TreatAsAtomicUnit=on
  If1 : If  NumInputs=2  IfExpression=u1 > u2 & u1 < 11000 & u1 >= 0
  Merge : Merge
  Merge1 : Merge
  Mux : Mux  Inputs=2
  Selector : Selector  InputPortWidth=2  IndexOptions=Index vector (dialog)  Indices=[1]  OutputSizes=1
  Selector1 : Selector  InputPortWidth=2  IndexOptions=Index vector (dialog)  Indices=[2]  OutputSizes=1
  newRange : Outport
  wires:
  Selector/1 -> If/2, If Action Subsystem1/1(In1)
  Selector1/1 -> If Action Subsystem3/1(In1), If1/2
  Mux/1 -> newRange/1
  Merge1/1 -> Mux/2
  Merge/1 -> Mux/1
  If Action Subsystem3/1(Out1) -> Merge1/2
  If Action Subsystem2/1(Out1) -> Merge1/1
  If1/2 -> If Action Subsystem3/Action
  If1/1 -> If Action Subsystem2/Action
  If Action Subsystem1/1(Out1) -> Merge/2
  If Action Subsystem/1(Out1) -> Merge/1
  If/2 -> If Action Subsystem1/Action
  If/1 -> If Action Subsystem/Action
  newValue/1 -> If Action Subsystem/1(In1), If/1, If Action Subsystem2/1(In1), If1/1
  limitRange/1 -> Selector/1, Selector1/1

== system code_gen_HeadingHold/Controller/Radio Control Inputs1/Calibration/Update range from input2 ==
  note: Update lower range limit.
      | The new value is checked against a sane range of 5000-11000
      | to keep values realistic.
  note: Update upper range limit
  limitRange : Inport
  newValue : Inport  Port=2
  If : If  NumInputs=2  IfExpression=u1 < u2 & u1 > 5000 & u1 >= 0
  If Action Subsystem : Subsystem  TreatAsAtomicUnit=on
  If Action Subsystem1 : Subsystem  TreatAsAtomicUnit=on
  If Action Subsystem2 : Subsystem  TreatAsAtomicUnit=on
  If Action Subsystem3 : Subsystem  TreatAsAtomicUnit=on
  If1 : If  NumInputs=2  IfExpression=u1 > u2 & u1 < 11000 & u1 >= 0
  Merge : Merge
  Merge1 : Merge
  Mux : Mux  Inputs=2
  Selector : Selector  InputPortWidth=2  IndexOptions=Index vector (dialog)  Indices=[1]  OutputSizes=1
  Selector1 : Selector  InputPortWidth=2  IndexOptions=Index vector (dialog)  Indices=[2]  OutputSizes=1
  newRange : Outport
  wires:
  Selector/1 -> If/2, If Action Subsystem1/1(In1)
  Selector1/1 -> If Action Subsystem3/1(In1), If1/2
  Mux/1 -> newRange/1
  Merge1/1 -> Mux/2
  Merge/1 -> Mux/1
  If Action Subsystem3/1(Out1) -> Merge1/2
  If Action Subsystem2/1(Out1) -> Merge1/1
  If1/2 -> If Action Subsystem3/Action
  If1/1 -> If Action Subsystem2/Action
  If Action Subsystem1/1(Out1) -> Merge/2
  If Action Subsystem/1(Out1) -> Merge/1
  If/2 -> If Action Subsystem1/Action
  If/1 -> If Action Subsystem/Action
  newValue/1 -> If Action Subsystem/1(In1), If/1, If Action Subsystem2/1(In1), If1/1
  limitRange/1 -> Selector/1, Selector1/1

== system code_gen_HeadingHold/Controller/Radio Control Inputs1/Detect calibration trigger/State outputs ==
  note: Define state outputs:
      | State 0: Not in calibration mode
      |   - LED is off
      | State 1: Calibration mode trigger test
      |   - LED is blinking at 10Hz
      | State 2: Calibration mode
      |   - LED is on
  cState : Inport
  If Action Subsystem1 : Subsystem  TreatAsAtomicUnit=on
  If Action Subsystem2 : Subsystem  TreatAsAtomicUnit=on
  If Action Subsystem3 : Subsystem  TreatAsAtomicUnit=on
  If Action Subsystem4 : Subsystem  TreatAsAtomicUnit=on
  If1 : If  IfExpression=u1 == 0 | u1 == 3  ElseIfExpressions=u1 == 1 | u1 == 4, u1 == 2
  Merge : Merge  Inputs=4  InitialOutput=false
  Rate Transition : RateTransition
  Repeating Sequence Stair : simulink/Sources/Repeating Sequence Stair  SystemSampleTime=-1  OutValues=[1 0]  tsamp=.1  OutMin=[]  OutMax=[]  OutDataTypeStr=fixdt('boolean')  OutputDataTypeScalingMode=Specify via dialog  OutDataType=fixdt('boolean')  ConRadixGroup=Best Precision: Vector-wise  OutScaling=[]
  LED : Outport
  wires:
  cState/1 -> If1/1
  Merge/1 -> LED/1
  If1/1 -> If Action Subsystem1/Action
  If1/2 -> If Action Subsystem3/Action
  If Action Subsystem1/1(LED) -> Merge/1
  If Action Subsystem3/1(LED) -> Merge/2
  If1/4 -> If Action Subsystem2/Action
  If1/3 -> If Action Subsystem4/Action
  If Action Subsystem4/1(LED) -> Merge/3
  If Action Subsystem2/1(LED) -> Merge/4
  Repeating Sequence Stair/1 -> Rate Transition/1
  Rate Transition/1 -> If Action Subsystem3/1(Pulse)

== system code_gen_HeadingHold/Controller/Radio Control Inputs1/If Action Subsystem1/Add 8% center deadband ==
  In1 : Inport
  If : If  IfExpression=u1 > -36 & u1 < 36
  If Action Subsystem : Subsystem  TreatAsAtomicUnit=on
  If Action Subsystem1 : Subsystem  TreatAsAtomicUnit=on
  Merge : Merge
  Out1 : Outport
  wires:
  In1/1 -> If Action Subsystem/1(In1), If/1
  If/2 -> If Action Subsystem/Action
  If/1 -> If Action Subsystem1/Action
  If Action Subsystem/1(Out1) -> Merge/2
  If Action Subsystem1/1(Out1) -> Merge/1
  Merge/1 -> Out1/1

== system code_gen_HeadingHold/Controller/Radio Control Inputs1/If Action Subsystem3/Add 5% deadband about 0 ==
  In1 : Inport
  If : If  IfExpression=u1 < 43 & u1 > -43
  If Action Subsystem : Subsystem  TreatAsAtomicUnit=on
  If Action Subsystem1 : Subsystem  TreatAsAtomicUnit=on
  Merge : Merge
  Out1 : Outport
  wires:
  In1/1 -> If Action Subsystem/1(In1), If/1
  If/2 -> If Action Subsystem/Action
  If/1 -> If Action Subsystem1/Action
  If Action Subsystem1/1(Out1) -> Merge/1
  Merge/1 -> Out1/1
  If Action Subsystem/1(Out1) -> Merge/2

== system code_gen_HeadingHold/Controller/Radio Control Inputs1/If Action Subsystem5/Add 8% center deadband ==
  In1 : Inport
  If : If  IfExpression=u1 > 460 & u1 < 540
  If Action Subsystem : Subsystem  TreatAsAtomicUnit=on
  If Action Subsystem1 : Subsystem  TreatAsAtomicUnit=on
  Merge : Merge
  Out1 : Outport
  wires:
  In1/1 -> If Action Subsystem/1(In1), If/1
  If/2 -> If Action Subsystem/Action
  If/1 -> If Action Subsystem1/Action
  If Action Subsystem/1(Out1) -> Merge/2
  If Action Subsystem1/1(Out1) -> Merge/1
  Merge/1 -> Out1/1

== system code_gen_HeadingHold/Controller/Split trackCommand to singular commands/Countdown timer for trigger/State transitions ==
  note: Define state transitions:
      | State 0: Not in calibration mode
      |   - Transition to state 1 if change
      | State 1: Transition trigger test
      |   - Transition to state 2 if level held
      |   - Transition to state 0 if level drops
      | State 2: Transition successful
      |   - Transition to state 0 if change
  timer : Inport
  level : Inport  Port=2
  timerState : Inport  Port=3
  If : If  NumInputs=3  IfExpression=u3 == 0 & u2 == 1  ElseIfExpressions=u3 == 1 & u2 == 0, u3 == 1 & u1 >= 100, u3 == 2 & u2 == 0
  Merge1 : Merge  Inputs=5  InitialOutput=false
  Merge2 : Merge  Inputs=5  InitialOutput=false
  Null transition (necessary for merge block) : Subsystem  TreatAsAtomicUnit=on
  Transition from 0 to 1 : Subsystem  TreatAsAtomicUnit=on
  Transition from 1 to 0 : Subsystem  TreatAsAtomicUnit=on
  Transition from 1 to 2 : Subsystem  TreatAsAtomicUnit=on
  Transition from 2 to 0 : Subsystem  TreatAsAtomicUnit=on
  startTimer : Outport
  trigger : Outport  Port=2
  wires:
  If/1 -> Transition from 0 to 1/Action
  If/5 -> Null transition (necessary for merge block)/Action
  timer/1 -> If/1
  timerState/1 -> If/3
  level/1 -> If/2
  If/2 -> Transition from 1 to 0/Action
  If/3 -> Transition from 1 to 2/Action
  If/4 -> Transition from 2 to 0/Action
  Merge1/1 -> startTimer/1
  Transition from 0 to 1/1(startTimer) -> Merge1/1
  Transition from 1 to 0/1(startTimer) -> Merge1/2
  Transition from 1 to 2/1(startTimer) -> Merge1/3
  Transition from 2 to 0/1(startTimer) -> Merge1/4
  Null transition (necessary for merge block)/1(startTimer) -> Merge1/5
  Merge2/1 -> trigger/1
  Transition from 0 to 1/2(trigger) -> Merge2/1
  Transition from 1 to 0/2(trigger) -> Merge2/2
  Transition from 1 to 2/2(trigger) -> Merge2/3
  Transition from 2 to 0/2(trigger) -> Merge2/4
  Null transition (necessary for merge block)/2(trigger) -> Merge2/5

== system code_gen_HeadingHold/Controller/Split trackCommand to singular commands/Countdown timer for trigger1/State transitions ==
  note: Define state transitions:
      | State 0: Not in calibration mode
      |   - Transition to state 1 if change
      | State 1: Transition trigger test
      |   - Transition to state 2 if level held
      |   - Transition to state 0 if level drops
      | State 2: Transition successful
      |   - Transition to state 0 if change
  timer : Inport
  level : Inport  Port=2
  timerState : Inport  Port=3
  If : If  NumInputs=3  IfExpression=u3 == 0 & u2 == 1  ElseIfExpressions=u3 == 1 & u2 == 0, u3 == 1 & u1 >= 100, u3 == 2 & u2 == 0
  Merge1 : Merge  Inputs=5  InitialOutput=false
  Merge2 : Merge  Inputs=5  InitialOutput=false
  Null transition (necessary for merge block) : Subsystem  TreatAsAtomicUnit=on
  Transition from 0 to 1 : Subsystem  TreatAsAtomicUnit=on
  Transition from 1 to 0 : Subsystem  TreatAsAtomicUnit=on
  Transition from 1 to 2 : Subsystem  TreatAsAtomicUnit=on
  Transition from 2 to 0 : Subsystem  TreatAsAtomicUnit=on
  startTimer : Outport
  trigger : Outport  Port=2
  wires:
  Null transition (necessary for merge block)/2(trigger) -> Merge2/5
  Transition from 2 to 0/2(trigger) -> Merge2/4
  Transition from 1 to 2/2(trigger) -> Merge2/3
  Transition from 1 to 0/2(trigger) -> Merge2/2
  Transition from 0 to 1/2(trigger) -> Merge2/1
  Merge2/1 -> trigger/1
  Null transition (necessary for merge block)/1(startTimer) -> Merge1/5
  Transition from 2 to 0/1(startTimer) -> Merge1/4
  Transition from 1 to 2/1(startTimer) -> Merge1/3
  Transition from 1 to 0/1(startTimer) -> Merge1/2
  Transition from 0 to 1/1(startTimer) -> Merge1/1
  Merge1/1 -> startTimer/1
  If/4 -> Transition from 2 to 0/Action
  If/3 -> Transition from 1 to 2/Action
  If/2 -> Transition from 1 to 0/Action
  level/1 -> If/2
  timerState/1 -> If/3
  timer/1 -> If/1
  If/5 -> Null transition (necessary for merge block)/Action
  If/1 -> Transition from 0 to 1/Action

== system code_gen_HeadingHold/Sensor Inputs/Estop detection/Receive ECAN1 Message/Decompose uint64 ==
  low-order uint32 : Inport  OutDataType=sfix(16)  OutScaling=2^0
  high-order uint1 : Inport  Port=2  OutDataType=sfix(16)  OutScaling=2^0
  Extract Bits : simulink/Logic and Bit Operations/Extract Bits  SystemSampleTime=-1  bitsToExtract=Range of bits  numBits=8  bitIdxRange=[0 7]  outScalingMode=Treat bit field as an integer
  Extract Bits1 : simulink/Logic and Bit Operations/Extract Bits  SystemSampleTime=-1  bitsToExtract=Range of bits  numBits=8  bitIdxRange=[8 15]  outScalingMode=Treat bit field as an integer
  Extract Bits2 : simulink/Logic and Bit Operations/Extract Bits  SystemSampleTime=-1  bitsToExtract=Range of bits  numBits=8  bitIdxRange=[16 23]  outScalingMode=Treat bit field as an integer
  Extract Bits3 : simulink/Logic and Bit Operations/Extract Bits  SystemSampleTime=-1  bitsToExtract=Range of bits  numBits=8  bitIdxRange=[24 31]  outScalingMode=Treat bit field as an integer
  Extract Bits4 : simulink/Logic and Bit Operations/Extract Bits  SystemSampleTime=-1  bitsToExtract=Range of bits  numBits=8  bitIdxRange=[0 7]  outScalingMode=Treat bit field as an integer
  Extract Bits5 : simulink/Logic and Bit Operations/Extract Bits  SystemSampleTime=-1  bitsToExtract=Range of bits  numBits=8  bitIdxRange=[8 15]  outScalingMode=Treat bit field as an integer
  Extract Bits6 : simulink/Logic and Bit Operations/Extract Bits  SystemSampleTime=-1  bitsToExtract=Range of bits  numBits=8  bitIdxRange=[16 23]  outScalingMode=Treat bit field as an integer
  Extract Bits7 : simulink/Logic and Bit Operations/Extract Bits  SystemSampleTime=-1  bitsToExtract=Range of bits  numBits=8  bitIdxRange=[24 31]  outScalingMode=Treat bit field as an integer
  Mux : Mux  Inputs=8
  uint8 array : Outport  OutDataType=sfix(16)  OutScaling=2^0
  wires:
  low-order uint32/1 -> Extract Bits/1, Extract Bits1/1, Extract Bits2/1, Extract Bits3/1
  Mux/1 -> uint8 array/1
  high-order uint1/1 -> Extract Bits4/1, Extract Bits5/1, Extract Bits6/1, Extract Bits7/1
  Extract Bits/1 -> Mux/1
  Extract Bits7/1 -> Mux/8
  Extract Bits1/1 -> Mux/2
  Extract Bits2/1 -> Mux/3
  Extract Bits3/1 -> Mux/4
  Extract Bits4/1 -> Mux/5
  Extract Bits5/1 -> Mux/6
  Extract Bits6/1 -> Mux/7

== system code_gen_HeadingHold/Controller/Auto/Manual Switch/Rudder calibration controller/Throttle Command/Mux Everything ==
  reset : Inport  OutDataType=sfix(16)  OutScaling=2^0
  0x300 : Constant  Value=768  OutDataTypeMode=uint32  OutDataType=sfix(16)  OutScaling=2^0  OutDataTypeStr=uint32
  Data Type Conversion1 : DataTypeConversion  OutDataTypeMode=boolean  OutDataType=sfix(16)  OutScaling=2^0  OutDataTypeStr=boolean
  Data Type Conversion3 : DataTypeConversion  OutDataTypeMode=boolean  OutDataType=sfix(16)  OutScaling=2^0  OutDataTypeStr=boolean
  Detect Change : simulink/Logic and Bit Operations/Detect Change  SystemSampleTime=-1  vinit=0
  Detect Rise Positive : simulink/Logic and Bit Operations/Detect Rise Positive  SystemSampleTime=-1  vinit=0
  Disable motor : Constant  Value=[0 0 0 0 64 0]  OutDataTypeMode=uint8  OutDataType=sfix(16)  OutScaling=2^0  OutDataTypeStr=uint8
  Enable motor : Constant  Value=[0 0 0 0 32 0]  OutDataTypeMode=uint8  OutDataType=sfix(16)  OutScaling=2^0  OutDataTypeStr=uint8
  Message Length1 : Probe  ProbeSampleTime=off  ProbeComplexSignal=off  ProbeWidthDataType=uint8
  Switch : Switch  Criteria=u2 ~= 0  OutDataType=fixdt(1, 16)  OutScaling=2^0
  iden : Outport  OutDataType=sfix(16)  OutScaling=2^0
  data : Outport  Port=2  OutDataType=sfix(16)  OutScaling=2^0
  size : Outport  Port=3  OutDataType=sfix(16)  OutScaling=2^0
  trig : Outport  Port=4  OutDataType=sfix(16)  OutScaling=2^0
  wires:
  0x300/1 -> iden/1
  Message Length1/1 -> size/1
  Switch/1 -> data/1, Message Length1/1
  Disable motor/1 -> Switch/1
  Enable motor/1 -> Switch/3
  Data Type Conversion1/1 -> Switch/2
  Detect Rise Positive/1 -> Data Type Conversion1/1
  reset/1 -> Detect Rise Positive/1, Detect Change/1
  Detect Change/1 -> Data Type Conversion3/1
  Data Type Conversion3/1 -> trig/1

== system code_gen_HeadingHold/Controller/Autonomous Controller/State Keeper & Estimator/GPS Estimator/Subsystem ==
  note: Multiply by .51444 to
      | convert knots to m/s
  gps : Inport
  Angle Conversion : uSimLib/Conversions/Angle Conversion  SystemSampleTime=-1  iu=deg  ou=rad
  Bus Selector : BusSelector  OutputSignals=sog
  Bus Selector1 : BusSelector  OutputSignals=cog
  Constant : Constant  Value=0  OutDataTypeMode=single  OutDataType=fixdt(1, 16)  OutScaling=2^0  OutDataTypeStr=single
  Gain : Gain  Gain=.5144444  ParameterDataType=fixdt(1, 16)  ParameterScaling=2^0  OutDataType=fixdt(1, 16)  OutScaling=2^0
  Mux : Mux  Inputs=3
  Product : Product  OutDataTypeMode=single  OutDataType=fixdt(1, 16)  OutScaling=2^0  OutDataTypeStr=single  RndMeth=Zero
  Product1 : Product  OutDataTypeMode=single  OutDataType=fixdt(1, 16)  OutScaling=2^0  OutDataTypeStr=single  RndMeth=Zero
  Reorder : Subsystem
  Trigonometric Function : Trigonometry
  Trigonometric Function1 : Trigonometry  Operator=cos
  velocity : Outport
  heading : Outport  Port=2
  pos : Outport  Port=3
  time : Outport  Port=4
  wires:
  Gain/1 -> Product1/1, Product/1
  gps/1 -> Reorder/1(In1), Bus Selector/1, Bus Selector1/1
  Bus Selector1/1 -> Angle Conversion/1  "<cog>"
  Trigonometric Function/1 -> Product/2
  Trigonometric Function1/1 -> Product1/2
  Product1/1 -> Mux/1
  Product/1 -> Mux/2
  Constant/1 -> Mux/3
  Mux/1 -> velocity/1
  Angle Conversion/1 -> heading/1, Trigonometric Function/1, Trigonometric Function1/1
  Bus Selector/1 -> Gain/1  "<sog>"
  Reorder/1(pos) -> pos/1
  Reorder/2(time) -> time/1
